simulink model "Modulation_Amplitude"  (R2023b)
settings: Solver=VariableStepAuto  StartTime=0.0  StopTime=10.0  RelTol=1e-3
settings Model: Creator=Spedrik Webster  LastModifiedBy=Spedrik Webster

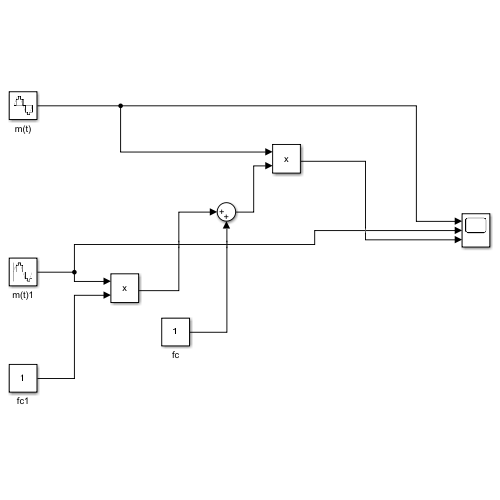
[thumbnail: Simulink's stored preview of the top-level diagram]
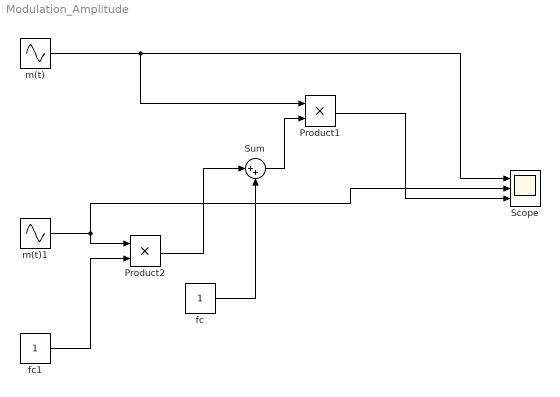
== system Modulation_Amplitude ==
  Product1 : Product
  Product2 : Product
  Scope : Scope  NumInputPorts=3
  Sum : Sum  Inputs=|++
  fc : Constant
  fc1 : Constant
  m(t) : Sin  Frequency=2  SampleTime=1/5000
  m(t)1 : Sin  Frequency=20  SampleTime=1/5000
  wires:
  fc/1 -> Sum/2
  Product2/1 -> Sum/1
  Sum/1 -> Product1/2
  m(t)/1 -> Product1/1, Scope/1
  m(t)1/1 -> Scope/2, Product2/1
  fc1/1 -> Product2/2
  Product1/1 -> Scope/3
